simulink model "difusop8"  (R2023a)
settings: Solver=VariableStepAuto  StartTime=0.0  StopTime=10.0  RelTol=1e-3
values from neighbouring files (symbols this model uses):
  A = [-1 1; 0 -2]    [punto8.m]
  B = [2;2]    [punto8.m]
  C = [1 2]    [punto8.m]
settings Model: Creator=mew-f  LastModifiedBy=mew-f

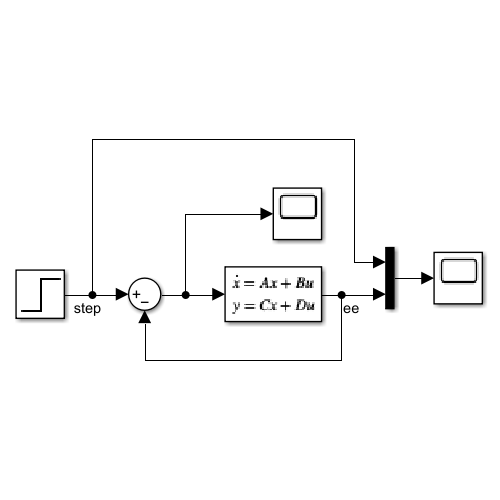
[thumbnail: Simulink's stored preview of the top-level diagram]
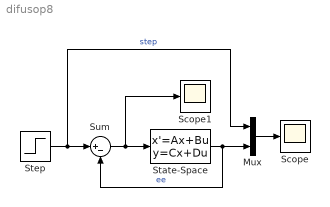
== system difusop8 ==
  Mux : Mux  Inputs=2
  Scope : Scope
  Scope1 : Scope
  State-Space : StateSpace  A=A  B=B  C=C  InitialCondition=0
  Step : Step  SampleTime=0
  Sum : Sum  Inputs=|+-
  wires:
  Mux/1 -> Scope/1
  State-Space/1 -> Sum/2, Mux/2  "ee"
  Step/1 -> Mux/1, Sum/1  "step"
  Sum/1 -> Scope1/1, State-Space/1
